simulink model "STmodel_gui"  (R2021b)
settings: Solver=FixedStepDiscrete  StartTime=0.0  StopTime=stop_time  FixedStep=Ts  MaxStep=Ts  RelTol=1e-6  EnableMultiTasking=on
PostLoadFcn:
  | , if any(exist('dsrtsu_mdlpostloadfcn', 'file') == [2, 3, 6]), try dsrtsu_mdlpostloadfcn('Execute', bdroot); catch fprintf('Error in PostLoadFcn (dsrtsu_mdlpostloadfcn) for model "%s":\n %s\n', bdroot, lasterr); end, end,
model workspace (MAT data in the model file):
  Tmp = Simulink.Parameter
  Tmp.Value = Simulink.data.Expression
  Tmp.Value.ExpressionString = "get_param(bdroot,'SimulationTime')"
  Tmp.DataType = 'auto'
  Tmp.Complexity = 'real'
  Tmp.Dimensions = -1
values from neighbouring files (symbols this model uses):
  Cf = 10e-6    (= 1e-05)    [init_STsetup.m]
  fc = 1/Ts    (= 1000)    [init_STsetup.m]
  Filter_d = c2d(Filter,Ts,'Tustin')    [init_STsetup.m]
  fref_st = 50    [init_STsetup.m]
  kii_ST = 250    [init_STsetup.m]
  kiv = 250    [init_STsetup.m]
  kpi_ST = 1.25    [init_STsetup.m]
  kpv = 0.2    [init_STsetup.m]
  Kqload = 2    [init_STsetup.m]
  Lc = 1e-3    (= 0.001)    [init_STsetup.m]
  LoadCurtailment = 0.9    [init_STsetup.m]
  LoadShedding = 0    [init_STsetup.m]
  log_time = 0.2    [init_STsetup.m]
  Pnom = 50e3    (= 50000)    [init_STsetup.m]
  Rc = 0.1    [init_STsetup.m]
  Rf = 2    [init_STsetup.m]
  STstartz = c2d(STstart,Ts,'Tustin')    [init_STsetup.m]
  Ts = 1e-3    (= 0.001)    [init_STsetup.m]
  Vdc = 650    [init_STsetup.m]
  Vref = 325    [init_STsetup.m]
undefined symbols (not defined in the file or in its folder): DiscIntNeverNeededParam
libraries: simulink x4, spsControlledVoltageSourceLib x3, spsThreePhaseSeriesRLCBranchLib x2, spsGroundLib x1, spsRMSLib x1, spsThreePhaseDynamicLoadLib x1, spsThreePhaseVIMeasurementLib x1, spspowerguiLib x1
(part 1 of 2)
settings Model: DSRTSU_INTERNAL_RTI_VER=480  DSRTSU_INTERNAL_RTI_TYPE=rti1006  DSRTSU_INTERNAL_RTIFPGA=70  TunableVars=COMP_GAIN,CurrentLoop,EN_AD,EN_COMPENSATION,EN_DG,EN_ST,FFselection,FREQ_ON,Iref,LEFcontrol,LoadCurtailment,LoadShedding,PLL_Tsettle,P_DG,Q_DG,RST_DG,RST_ST,RSTanalog,VARF,VARV,Vref,calibrationDC_en,calibration_en,fref_st,kc,kii,kii_ST,kiv,kpi,kpi_ST,kpv,krci,krcv,krv  TunableVarsStorageClass=Auto,Auto,Auto,Auto,Auto,Auto,Auto,Auto,Auto,Auto,Auto,Auto,Auto,Auto,Auto,Auto,Auto,Auto,Auto,Auto,Auto,Auto,Auto,Auto,Auto,Auto,Auto,Auto,Auto,Auto,Auto,Auto,Auto,Auto  TunableVarsTypeQualifier=,,,,,,,,,,,,,,,,,,,,,,,,,,,,,,,,,  Creator=zz  LastModifiedBy=bela
settings SolverCC: ConcurrentTasks=on  AlgebraicLoopSolver=TrustRegion  AutoInsertRateTranBlk=on
settings DataIOCC: LimitDataPoints=on  SaveFormat=StructureWithTime  ReturnWorkspaceOutputs=off
settings OptimizationCC: BlockReduction=off  DefaultParameterBehavior=Inlined  EnhancedBackFolding=on  PassReuseOutputArgsAs=Individual arguments  ZeroExternalMemoryAtStartup=off  ZeroInternalMemoryAtStartup=off  OptimizeBlockOrder=speed  DifferentSizesBufferReuse=on  OptimizationCustomize=off  EfficientTunableParamExpr=on
settings DebuggingCC: SolverPrmCheckMsg=warning  ParameterTunabilityLossMsg=error  SFUnexpectedBacktrackingDiag=warning  SFNoUnconditionalDefaultTransitionDiag=warning  SFMachineParentedDataDiag=warning  ArithmeticOperatorsInVariantConditions=warning
settings HardwareCC: ProdBitPerPointer=32  ProdBitPerSizeT=32  ProdBitPerPtrDiffT=32  ProdLargestAtomicFloat=None  ProdWordSize=32  ProdLongLongMode=on  ProdHWDeviceType=Generic->32-bit x86 compatible  TargetBitPerLong=64  TargetBitPerPointer=64  TargetBitPerSizeT=64  TargetBitPerPtrDiffT=64  TargetLongLongMode=on  TargetIntDivRoundTo=Zero  TargetEndianess=LittleEndian  TargetWordSize=64  TargetHWDeviceType=MATLAB Host  ProdEqTarget=off
settings ModelReferenceCC: PropagateSignalLabelsOutOfModel=off
settings SFSimCC: SimUseLocalCustomCode=off  MATLABDynamicMemAlloc=off  CustomCodeUndefinedFunction=UseInterfaceOnly
settings RTWCC: Description=Embedded Coder  SystemTargetFile=ert.tlc  TemplateMakefile=ert_default_tmf  RTWUseLocalCustomCode=off  CodeExecutionProfiling=on  RTWCompilerOptimization=on  CheckMdlBeforeBuild=Warning
settings CodeAppCC: ForceParamTrailComments=on  IgnoreCustomStorageClasses=off  OperatorAnnotations=on  SimulinkDataObjDesc=on  SFDataObjDesc=on  InsertBlockDesc=on
settings ERTTargetCC: TargetLangStandard=C99 (ISO)  GenerateSampleERTMain=on  SupportNonInlinedSFcns=on  InlinedParameterPlacement=NonHierarchical  TargetOS=NativeThreadsExample  ERTCustomFileTemplate=example_file_process.tlc
settings ConfigComp: CovMetricSettings=dw  CovSaveCumulativeToWorkspaceVar=on  CovSaveSingleToWorkspaceVar=on  CovExternalEMLEnable=off  CovSFcnEnable=off

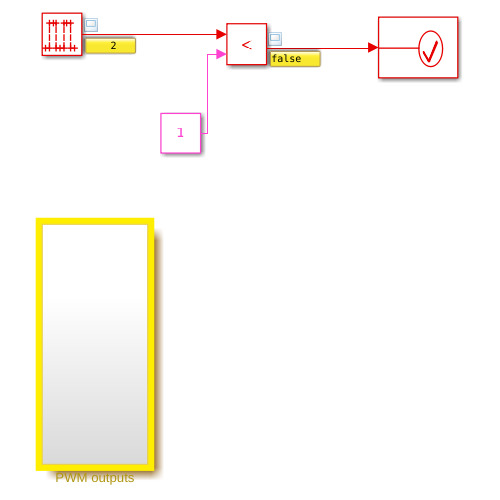
[thumbnail: Simulink's stored preview of the top-level diagram]
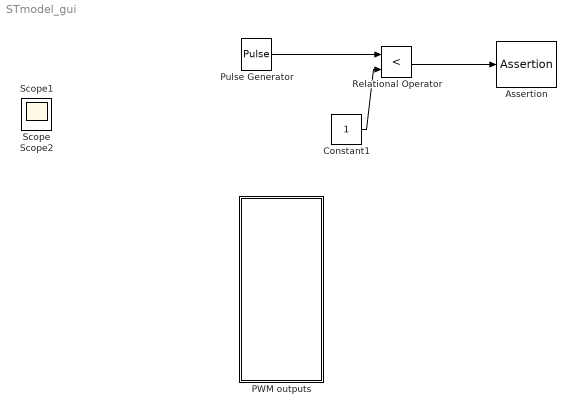
== system STmodel_gui ==
  Assertion : Assertion  AssertionFailFcn=set_param(bdroot,'SimulationCommand','pause')  StopWhenAssertionFail=off
  Constant1 : Constant
  PWM outputs : Subsystem
  Pulse Generator : DiscretePulseGenerator  Amplitude=2  Period=floor(log_time/Ts)  SampleTime=Ts
  Relational Operator : RelationalOperator  Operator=<  OutDataTypeStr=boolean  RndMeth=Simplest
  Scope : Scope
  Scope1 : Scope
  Scope2 : Scope
  wires:
  Constant1/1 -> Relational Operator/2
  Relational Operator/1 -> Assertion/1
  Pulse Generator/1 -> Relational Operator/1

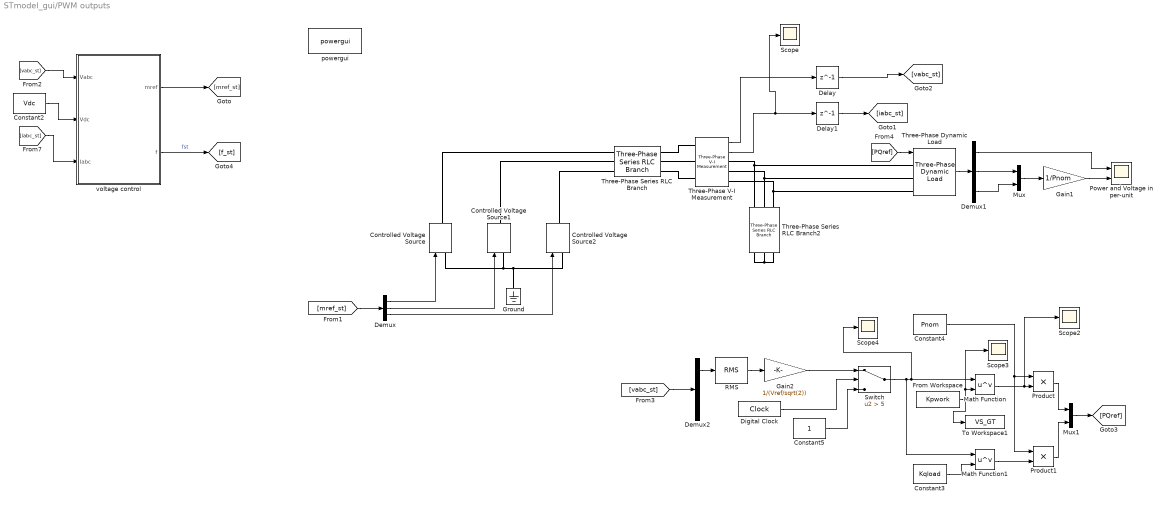
== system STmodel_gui/PWM outputs ==
  Constant2 : Constant  Value=Vdc
  Constant3 : Constant  Value=Kqload
  Constant4 : Constant  Value=Pnom
  Constant5 : Constant
  Controlled Voltage Source : spsControlledVoltageSourceLib/Controlled Voltage Source  Initialize=on  Source_Type=AC  Amplitude=0  Phase=0  Frequency=0  Measurements=None
  Controlled Voltage Source1 : spsControlledVoltageSourceLib/Controlled Voltage Source  Initialize=on  Source_Type=AC  Amplitude=0  Phase=0  Frequency=0  Measurements=None
  Controlled Voltage Source2 : spsControlledVoltageSourceLib/Controlled Voltage Source  Initialize=on  Source_Type=AC  Amplitude=0  Phase=0  Frequency=0  Measurements=None
  Delay : Delay  DelayLength=1  InitialCondition=0
  Delay1 : Delay  DelayLength=1  InitialCondition=0
  Demux : Demux  Outputs=3
  Demux1 : Demux  Outputs=3
  Demux2 : Demux  Outputs=3
  Digital Clock : DigitalClock  SampleTime=Ts
  From Workspace : FromWorkspace  VariableName=Kpwork  OutDataTypeStr=double  SampleTime=-1
  Gain1 : Gain  Gain=1/Pnom
  Gain2 : Gain  Gain=1/(Vref/sqrt(2))
  Ground : spsGroundLib/Ground  LConnTagsString=a
  Math Function : Math  Operator=pow  SaturateOnIntegerOverflow=on
  Math Function1 : Math  Operator=pow  SaturateOnIntegerOverflow=on
  Mux : Mux  Inputs=2
  Mux1 : Mux  Inputs=2
  Power and Voltage in per-unit : Scope  NumInputPorts=2
  Product : Product
  Product1 : Product
  RMS : spsRMSLib/RMS  TrueRMS=on  Freq=50  RMSInit=230  Ts=Ts
  Scope{,2..4} (4 alike) : Scope
  Switch : Switch  Criteria=u2 > Threshold  Threshold=5
  Three-Phase Dynamic Load : spsThreePhaseDynamicLoadLib/Three-Phase Dynamic Load  NominalVoltage=[ 325/sqrt(2)*sqrt(3) 50 ]  ActiveReactivePowers=[50e3 0]  PositiveSequence=[1 0]  ExternalControl=on  NpNq=[1.3 2]  TimeConstants="[0  0  0  0]"  MinimumVoltage=0.7  Tfilter=1e-4  LoadFlowParameters=[4,0,0,0,0]
      settings: SourceProductBaseCode=PS
  Three-Phase Series RLC Branch : spsThreePhaseSeriesRLCBranchLib/Three-Phase Series RLC Branch  LConnTagsString=A|B|C  RConnTagsString=A|B|C  BranchType=RL  Resistance=Rc  Inductance=Lc  Capacitance=1e-6  Measurements=None
  Three-Phase Series RLC Branch2 : spsThreePhaseSeriesRLCBranchLib/Three-Phase Series RLC Branch  LConnTagsString=A|B|C  RConnTagsString=A|B|C  BranchType=RC  Resistance=Rf  Inductance=Lc  Capacitance=Cf  Measurements=None
  Three-Phase V-I Measurement : spsThreePhaseVIMeasurementLib/Three-Phase V-I Measurement  VoltageMeasurement=phase-to-ground  SetLabelV=off  LabelV=Vabc  Vpu=off  VpuLL=off  CurrentMeasurement=yes  SetLabelI=off  LabelI=Iabc  Ipu=off  Pbase=100e6  Vbase=Vref*sqrt(3)/sqrt(2)  OutputType=Complex  PhasorSimulation=off  PSBequivalent=0
  To Workspace1 : ToWorkspace  VariableName=VS_GT  SampleTime=log_time
      settings: MaxDataPoints=floor(log_time/Ts)  Save2DSignal=2-D array (concatenate along first dimension)
  powergui : spspowerguiLib/powergui  Priority=1  SimulationMode=Discrete  SampleTime=Ts  frequency=60  Iterations=50  frequencyindice=0  Pbase=100e6  ErrMax=1e-4  UnitsV=kV  UnitsW=MW  buscounter=0  FunctionMessages=off  echomessages=off  EnableUseOfTLC=off  CurrentSourceSwitches=off  DisableSnubberDevices=off  DisableRonSwitches=off  DisableVfSwitches=off  DisplayEquations=off  AutomaticDiscreteSolvers=off  SolverType=Tustin/Backward Euler (TBE)  Interpol=off  ExternalGateDelay=off  methode=off  Ts=100  x0status=blocks  SPID=on  SwTol=0  HookPort=off  NonlinearTolerance=1e-4  nMaxIteration=100  ContinueOnMaxIteration=off  RestoreLinks=warning  ResistiveCurrentMeasurement=off  Frange=[0:2:500]  Ylog=off  Xlog=on  ShowGrid=off  save=off  variable=ZData  structure=0  ZoomFFT=off  StartTime=0.0  cycles=1  DisplayStyle=1  fundamental=60  FreqAxis=off  MaxFrequency=1000  frequencyindicesteady=1  RmsSteady=1  display=off
  voltage control : Subsystem
  wires:
  voltage control/1(mref) -> [mref_st]
  [vabc_st] -> voltage control/1(Vabc)
  Constant2/1 -> voltage control/2(Vdc)
  [iabc_st] -> voltage control/3(Iabc)
  voltage control/2(f) -> [f_st]  "fst"
  [mref_st] -> Demux/1
  Demux/3 -> Controlled Voltage Source2/1
  Demux/2 -> Controlled Voltage Source1/1
  Demux/1 -> Controlled Voltage Source/1
  Three-Phase V-I Measurement/2 -> Scope/1, Delay1/1
  Three-Phase V-I Measurement/1 -> Delay/1
  Delay/1 -> [vabc_st]
  Delay1/1 -> [iabc_st]
  Demux1/1 -> Power and Voltage in per-unit/1
  Demux1/2 -> Mux/1
  Demux1/3 -> Mux/2
  Mux/1 -> Gain1/1
  Gain1/1 -> Power and Voltage in per-unit/2
  RMS/1 -> Gain2/1
  Switch/1 -> Math Function1/1, Scope4/1, Math Function/1
  From Workspace/1 -> To Workspace1/1, Scope3/1, Math Function/2
  Constant3/1 -> Math Function1/2
  Math Function/1 -> Scope2/1, Product/2
  Math Function1/1 -> Product1/2
  Constant4/1 -> Product1/1, Product/1
  Mux1/1 -> [PQref]
  Product/1 -> Mux1/1
  Product1/1 -> Mux1/2
  [vabc_st] -> Demux2/1
  Gain2/1 -> Switch/1
  Constant5/1 -> Switch/3
  Digital Clock/1 -> Switch/2
  Three-Phase Dynamic Load/1 -> Demux1/1
  [PQref] -> Three-Phase Dynamic Load/1
  Demux2/1 -> RMS/1
  connections:
  Controlled Voltage Source/LConn1 -- Ground/LConn1 -- Controlled Voltage Source2/LConn1 -- Controlled Voltage Source1/LConn1
  Three-Phase Series RLC Branch2/RConn1 -- Three-Phase Series RLC Branch2/RConn3 -- Three-Phase Series RLC Branch2/RConn2
  Three-Phase Series RLC Branch/LConn1 -- Controlled Voltage Source/RConn1
  Three-Phase Series RLC Branch/LConn2 -- Controlled Voltage Source1/RConn1
  Three-Phase Series RLC Branch/LConn3 -- Controlled Voltage Source2/RConn1
  Three-Phase V-I Measurement/LConn2 -- Three-Phase Series RLC Branch/RConn2
  Three-Phase Series RLC Branch/RConn1 -- Three-Phase V-I Measurement/LConn1
  Three-Phase Series RLC Branch/RConn3 -- Three-Phase V-I Measurement/LConn3
  Three-Phase V-I Measurement/RConn1 -- Three-Phase Dynamic Load/LConn1 -- Three-Phase Series RLC Branch2/LConn1
  Three-Phase V-I Measurement/RConn2 -- Three-Phase Dynamic Load/LConn2 -- Three-Phase Series RLC Branch2/LConn2
  Three-Phase V-I Measurement/RConn3 -- Three-Phase Dynamic Load/LConn3 -- Three-Phase Series RLC Branch2/LConn3

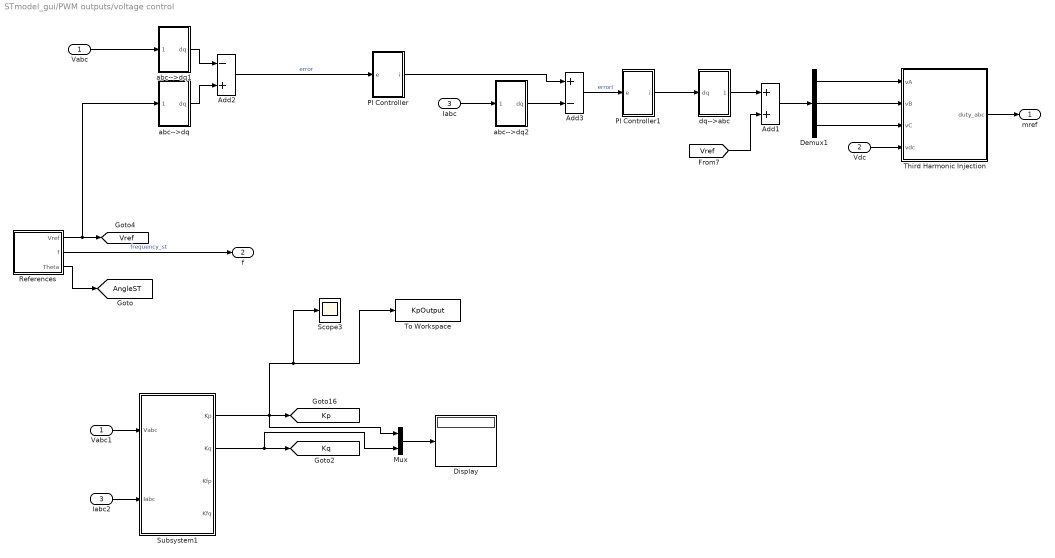
== system STmodel_gui/PWM outputs/voltage control ==
  Vabc : Inport
  Vdc : Inport  Port=2
  Iabc : Inport  Port=3
  Add1 : Sum
  Add2 : Sum  Inputs=-+
  Add3 : Sum  Inputs=+-
  Demux1 : Demux  Outputs=3
  Display : Display
  Iabc2 : InportShadow  Port=3
  Mux : Mux  Inputs=2
  PI Controller : Subsystem
  PI Controller1 : Subsystem
  References : Subsystem
  Scope3 : Scope
  Subsystem1 : Subsystem
  Third Harmonic Injection : Subsystem
      mask Display: disp('Modulation');
  To Workspace : ToWorkspace  VariableName=KpOutput  SampleTime=log_time
      settings: MaxDataPoints=floor(log_time/Ts)  Save2DSignal=2-D array (concatenate along first dimension)
  Vabc1 : InportShadow
  abc-->dq : Subsystem
  abc-->dq1 : Subsystem
  abc-->dq2 : Subsystem
  dq-->abc : Subsystem
  mref : Outport
  f : Outport  Port=2
  tag scope: AngleST=global, Kp=global, Kq=global, Vref=global
  wires:
  [Vref] -> Add1/2
  Vabc1/1 -> Subsystem1/1(Vabc)
  Iabc2/1 -> Subsystem1/2(Iabc)
  Subsystem1/2(Kq) -> Mux/2, [Kq]
  Subsystem1/1(Kp) -> Scope3/1, To Workspace/1, Mux/1, [Kp]
  Demux1/3 -> Third Harmonic Injection/3(vC)
  Demux1/2 -> Third Harmonic Injection/2("vB ")
  Demux1/1 -> Third Harmonic Injection/1(vA)
  Add2/1 -> PI Controller/1(e)  "error"
  Vabc/1 -> abc-->dq1/1(abc)
  References/2(f) -> f/1  "frequency_st"
  References/1(Vref) -> abc-->dq/1(abc), [Vref]
  Vdc/1 -> Third Harmonic Injection/4(vdc)
  Third Harmonic Injection/1(duty_abc) -> mref/1
  Iabc/1 -> abc-->dq2/1(abc)
  Add3/1 -> PI Controller1/1(e)  "errorI"
  abc-->dq2/1(dq) -> Add3/2
  References/3(Theta) -> [AngleST]
  abc-->dq/1(dq) -> Add2/2
  abc-->dq1/1(dq) -> Add2/1
  PI Controller1/1(i) -> dq-->abc/1(dq)
  dq-->abc/1(abc) -> Add1/1
  PI Controller/1(i) -> Add3/1
  Mux/1 -> Display/1
  Add1/1 -> Demux1/1

== system STmodel_gui/PWM outputs/voltage control/PI Controller ==
  e : Inport
  Demux : Demux  Outputs=2
  Mux1 : Mux  Inputs=2
  Subsystem1 : Subsystem
  Subsystem2 : Subsystem
  i : Outport
  wires:
  Mux1/1 -> i/1
  Subsystem2/1(out) -> Mux1/2
  Subsystem1/1(out) -> Mux1/1
  Demux/2 -> Subsystem2/1(e)
  Demux/1 -> Subsystem1/1(e)
  e/1 -> Demux/1

== system STmodel_gui/PWM outputs/voltage control/PI Controller1 ==
  e : Inport
  Demux : Demux  Outputs=2
  Mux1 : Mux  Inputs=2
  Subsystem1 : Subsystem
  Subsystem2 : Subsystem
  i : Outport
  wires:
  e/1 -> Demux/1
  Demux/1 -> Subsystem1/1(e)
  Demux/2 -> Subsystem2/1(e)
  Subsystem1/1(out) -> Mux1/1
  Subsystem2/1(out) -> Mux1/2
  Mux1/1 -> i/1

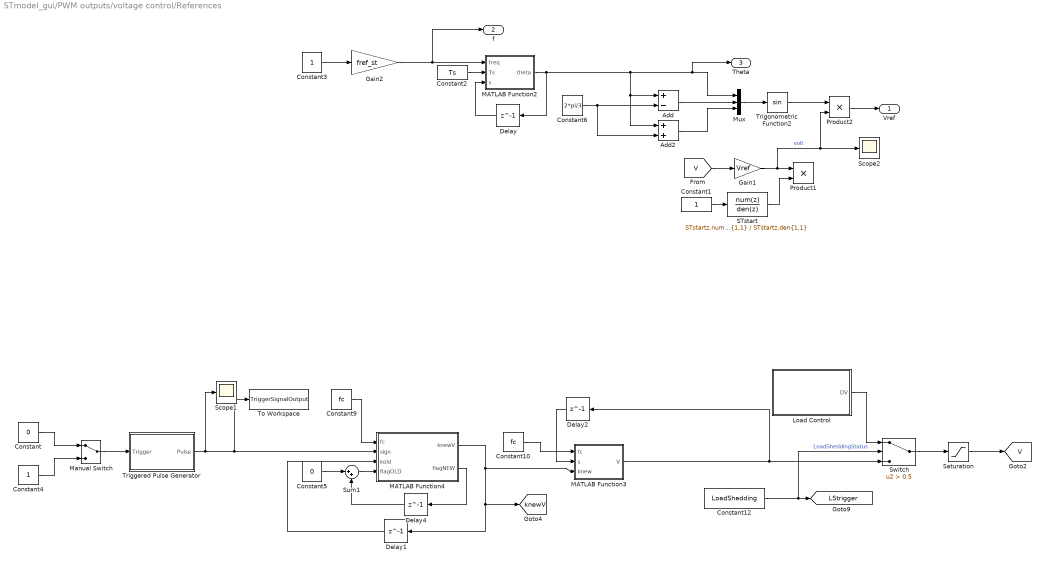
== system STmodel_gui/PWM outputs/voltage control/References ==
  Add : Sum  Inputs=+-
  Add2 : Sum
  Constant : Constant  Value=0
  Constant1 : Constant
  Constant10 : Constant  Value=fc
  Constant12 : Constant  Value=LoadShedding
  Constant2 : Constant  Value=Ts
  Constant3 : Constant
  Constant4 : Constant
  Constant5 : Constant  Value=0
  Constant6 : Constant  Value=2*pi/3
  Constant9 : Constant  Value=fc
  Delay{,1..2,4} (4 alike) : Delay  DelayLength=1  InitialCondition=0
  Gain1 : Gain  Gain=Vref
  Gain2 : Gain  Gain=fref_st
  Load Control : Subsystem
  MATLAB Function2 : MATLAB Function  TreatAsAtomicUnit=on
  MATLAB Function3 : MATLAB Function  TreatAsAtomicUnit=on
  MATLAB Function4 : MATLAB Function  TreatAsAtomicUnit=on
  Manual Switch : ManualSwitch
  Mux : Mux  Inputs=3
  Product1 : Product
  Product2 : Product
  STstart : DiscreteFilter  Numerator=STstartz.num{1,1}  Denominator=STstartz.den{1,1}
  Saturation : Saturate  UpperLimit=1.1  LowerLimit=0.85
  Scope1 : Scope
  Scope2 : Scope
  Sum1 : Sum  Inputs=|++
  Switch : Switch  Criteria=u2 > Threshold  Threshold=0.5
  To Workspace : ToWorkspace  VariableName=TriggerSignalOutput  SampleTime=log_time
      settings: MaxDataPoints=floor(log_time/Ts)  Save2DSignal=2-D array (concatenate along first dimension)
  Triggered Pulse Generator : Subsystem  TreatAsAtomicUnit=on  mask(single pulse generation){p_wid=2000}
      mask prompts: p_wid "pulse width (number of samples)"
      mask help: This block generate a single pulse whenever a trigger happen. The pulse width must specified as a number of samples. for example if your sampling time is 0.1s and you want 3s pulse , then you should enter 30 as a pulse width.
      mask Display:
      | plot([0],[0])
      | plot([11],[0])
      | plot([5],[0.5])
      | plot([4 5 5 6 6 7],[0 0 0.25 0.25 0 0])
      | plot([5],[-0.3])
      | 
      | port_label('output', 1, 'Pulse')
      | port_label('input', 1, 'Trigger')
  Trigonometric Function2 : Trigonometry
  Vref : Outport
  f : Outport  Port=2
  Theta : Outport  Port=3
  tag scope: LStrigger=global, V=global, knewV=global
  wires:
  Saturation/1 -> [V]
  Switch/1 -> Saturation/1
  MATLAB Function3/1(V) -> Switch/3, Delay2/1
  Constant12/1 -> [LStrigger], Switch/2  "LoadSheddingStatus"
  Constant10/1 -> MATLAB Function3/1(fc)
  Constant9/1 -> MATLAB Function4/1(fc)
  Delay4/1 -> Sum1/2
  MATLAB Function4/2(flagNEW) -> Delay4/1
  Sum1/1 -> MATLAB Function4/4(flagOLD)
  Constant5/1 -> Sum1/1
  Delay1/1 -> MATLAB Function4/3(kold)
  MATLAB Function4/1(knewV) -> MATLAB Function3/3(knew), Delay1/1, [knewV]
  Delay2/1 -> MATLAB Function3/2(s)
  Product2/1 -> Vref/1
  Mux/1 -> Trigonometric Function2/1
  MATLAB Function2/1(theta) -> Theta/1, Mux/1, Add/1, Add2/1, Delay/1
  Constant6/1 -> Add2/2, Add/2
  Add/1 -> Mux/2
  Add2/1 -> Mux/3
  Delay/1 -> MATLAB Function2/3(s)
  Trigonometric Function2/1 -> Product2/1
  Gain2/1 -> MATLAB Function2/1(freq), f/1
  [V] -> Gain1/1
  Constant3/1 -> Gain2/1
  Constant2/1 -> MATLAB Function2/2(Ts)
  Gain1/1 -> Scope2/1, Product2/2, Product1/1  "volt"
  Constant1/1 -> STstart/1
  STstart/1 -> Product1/2
  Load Control/1(DV) -> Switch/1
  Constant4/1 -> Manual Switch/2
  Constant/1 -> Manual Switch/1
  Manual Switch/1 -> Triggered Pulse Generator/1(Trigger)
  Triggered Pulse Generator/1(Pulse) -> Scope1/1, MATLAB Function4/2(sign), To Workspace/1

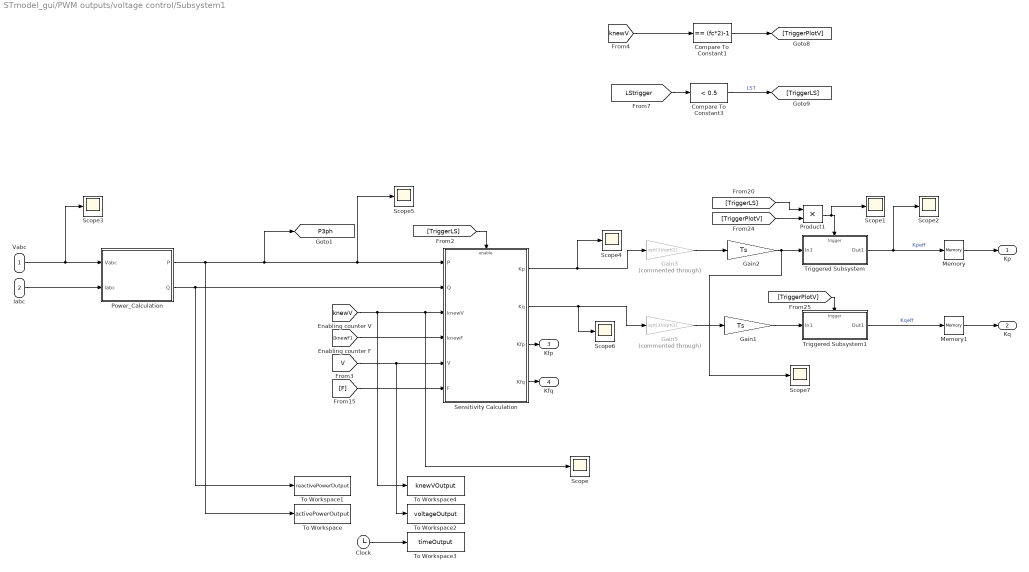
== system STmodel_gui/PWM outputs/voltage control/Subsystem1 ==
  Vabc : Inport
  Iabc : Inport  Port=2
  Clock : Clock
  Compare To Constant1 : simulink/Logic and Bit Operations/Compare To Constant  relop===  const=(fc*2)-1  OutDataTypeStr=boolean
  Compare To Constant3 : simulink/Logic and Bit Operations/Compare To Constant  relop=<  const=0.5  OutDataTypeStr=boolean
  Gain1 : Gain  Gain=Ts
  Gain2 : Gain  Gain=Ts
  Gain3 : Gain  Commented=through  Gain=sqrt(3)/sqrt(2)
  Gain5 : Gain  Commented=through  Gain=sqrt(3)/sqrt(2)
  Memory : Memory  InitialCondition=1  InheritSampleTime=on
  Memory1 : Memory  InheritSampleTime=on
  Power_Calculation : Subsystem
  Product1 : Product
  Scope{,1..7} (8 alike) : Scope
  Sensitivity Calculation : Subsystem  TreatAsAtomicUnit=on
  To Workspace : ToWorkspace  VariableName=activePowerOutput  SampleTime=log_time
      settings: MaxDataPoints=floor(log_time/Ts)  Save2DSignal=2-D array (concatenate along first dimension)
  To Workspace1 : ToWorkspace  VariableName=reactivePowerOutput  SampleTime=log_time
      settings: MaxDataPoints=floor(log_time/Ts)  Save2DSignal=2-D array (concatenate along first dimension)
  To Workspace2 : ToWorkspace  VariableName=voltageOutput  SampleTime=log_time
      settings: MaxDataPoints=floor(log_time/Ts)  Save2DSignal=2-D array (concatenate along first dimension)
  To Workspace3 : ToWorkspace  VariableName=timeOutput  SampleTime=log_time
      settings: MaxDataPoints=floor(log_time/Ts)  Save2DSignal=2-D array (concatenate along first dimension)
  To Workspace4 : ToWorkspace  VariableName=knewVOutput  SampleTime=log_time
      settings: MaxDataPoints=floor(log_time/Ts)  Save2DSignal=2-D array (concatenate along first dimension)
  Triggered Subsystem : Subsystem  TreatAsAtomicUnit=on
  Triggered Subsystem1 : Subsystem  TreatAsAtomicUnit=on
  Kp : Outport
  Kq : Outport  Port=2
  Kfp : Outport  Port=3
  Kfq : Outport  Port=4
  tag scope: P3ph=global
  wires:
  Sensitivity Calculation/4(Kfq) -> Kfq/1
  Sensitivity Calculation/3(Kfp) -> Kfp/1
  Gain2/1 -> Scope7/1, Triggered Subsystem/1(In1)
  [TriggerPlotV] -> Triggered Subsystem1/Trigger
  Triggered Subsystem/1(Out1) -> Scope2/1, Memory/1  "Kpeff"
  Triggered Subsystem1/1(Out1) -> Memory1/1  "Kqeff"
  Gain1/1 -> Triggered Subsystem1/1(In1)
  Sensitivity Calculation/2(Kq) -> Scope6/1, Gain5/1
  [knewV] -> Compare To Constant1/1
  Compare To Constant1/1 -> [TriggerPlotV]
  [knewV] -> To Workspace4/1, Scope/1, Sensitivity Calculation/3(knewV)
  [knewF] -> Sensitivity Calculation/4(knewF)
  [V] -> To Workspace2/1, Sensitivity Calculation/5(V)
  [F] -> Sensitivity Calculation/6(F)
  Memory/1 -> Kp/1
  [LStrigger] -> Compare To Constant3/1
  Compare To Constant3/1 -> [TriggerLS]  "LST"
  [TriggerLS] -> Sensitivity Calculation/Enable
  [TriggerPlotV] -> Product1/2
  [TriggerLS] -> Product1/1
  Product1/1 -> Scope1/1, Triggered Subsystem/Trigger
  Memory1/1 -> Kq/1
  Power_Calculation/1(P) -> To Workspace/1, Sensitivity Calculation/1(P), Scope5/1, [P3ph]
  Vabc/1 -> Scope3/1, Power_Calculation/1(Vabc)
  Iabc/1 -> Power_Calculation/2(Iabc)
  Gain3/1 -> Gain2/1
  Gain5/1 -> Gain1/1
  Power_Calculation/2(Q) -> To Workspace1/1, Sensitivity Calculation/2(Q)
  Clock/1 -> To Workspace3/1
  Sensitivity Calculation/1(Kp) -> Scope4/1, Gain3/1

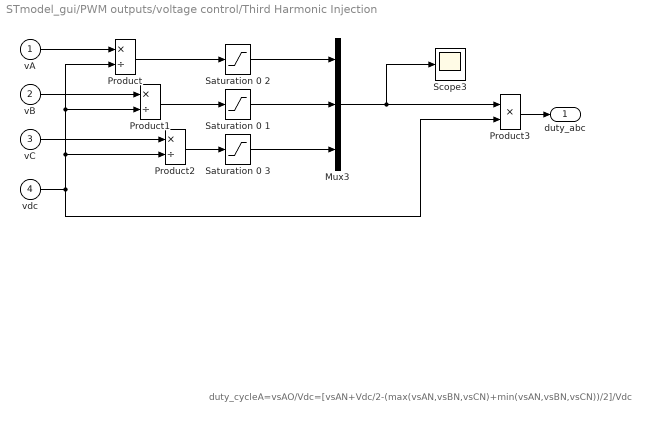
== system STmodel_gui/PWM outputs/voltage control/Third Harmonic Injection ==
  note: duty_cycleA=vsAO/Vdc=[vsAN+Vdc/2-(max(vsAN,vsBN,vsCN)+min(vsAN,vsBN,vsCN))/2]/Vdc
  vA : Inport
  "vB " : Inport  Port=2
  vC : Inport  Port=3
  vdc : Inport  Port=4
  Mux3 : Mux  Inputs=3
  Product : Product  Inputs=*/  SaturateOnIntegerOverflow=on  OutDataTypeStr=Inherit: Same as first input
  Product1 : Product  Inputs=*/  SaturateOnIntegerOverflow=on  OutDataTypeStr=Inherit: Same as first input
  Product2 : Product  Inputs=*/  SaturateOnIntegerOverflow=on  OutDataTypeStr=Inherit: Same as first input
  Product3 : Product  Inputs=**  SaturateOnIntegerOverflow=on  OutDataTypeStr=Inherit: Same as first input
  Saturation 0 1 : Saturate  UpperLimit=1  LowerLimit=-1
  Saturation 0 2 : Saturate  UpperLimit=1  LowerLimit=-1
  Saturation 0 3 : Saturate  UpperLimit=1  LowerLimit=-1
  Scope3 : Scope
  duty_abc : Outport
  wires:
  Product2/1 -> Saturation 0 3/1
  "vB "/1 -> Product1/1
  vdc/1 -> Product3/2, Product2/2, Product1/2, Product/2
  Product1/1 -> Saturation 0 1/1
  Product/1 -> Saturation 0 2/1
  Saturation 0 3/1 -> Mux3/3
  Saturation 0 1/1 -> Mux3/2
  Saturation 0 2/1 -> Mux3/1
  vA/1 -> Product/1
  vC/1 -> Product2/1
  Mux3/1 -> Scope3/1, Product3/1
  Product3/1 -> duty_abc/1

== system STmodel_gui/PWM outputs/voltage control/abc-->dq ==
  abc : Inport
  alpha,beta --> d,q1 : Subsystem
  clarke3 : Gain  Gain=(2/3)*[1 -0.5 -0.5; 0 sqrt(3)/2 -sqrt(3)/2]  Multiplication=Matrix(K*u)
  dq : Outport
  wires:
  alpha,beta --> d,q1/1(d,q) -> dq/1
  clarke3/1 -> alpha,beta --> d,q1/1("alpha, beta")
  [AngleST] -> alpha,beta --> d,q1/2(phi)
  abc/1 -> clarke3/1

== system STmodel_gui/PWM outputs/voltage control/abc-->dq1 ==
  abc : Inport
  alpha,beta --> d,q : Subsystem
  clarke2 : Gain  Gain=(2/3)*[1 -0.5 -0.5; 0 sqrt(3)/2 -sqrt(3)/2]  Multiplication=Matrix(K*u)
  dq : Outport
  wires:
  alpha,beta --> d,q/1(d,q) -> dq/1  "vref"
  clarke2/1 -> alpha,beta --> d,q/1("alpha, beta")  "vref"
  [AngleST] -> alpha,beta --> d,q/2(phi)
  abc/1 -> clarke2/1

== system STmodel_gui/PWM outputs/voltage control/abc-->dq2 ==
  abc : Inport
  alpha,beta --> d,q1 : Subsystem
  clarke3 : Gain  Gain=(2/3)*[1 -0.5 -0.5; 0 sqrt(3)/2 -sqrt(3)/2]  Multiplication=Matrix(K*u)
  dq : Outport
  wires:
  abc/1 -> clarke3/1
  [AngleST] -> alpha,beta --> d,q1/2(phi)
  clarke3/1 -> alpha,beta --> d,q1/1("alpha, beta")
  alpha,beta --> d,q1/1(d,q) -> dq/1

== system STmodel_gui/PWM outputs/voltage control/dq-->abc ==
  dq : Inport
  alpha,beta --> d,q3 : Subsystem
  clarke : Gain  Gain=[1 0; -0.5 sqrt(3)/2; -0.5 -sqrt(3)/2]  Multiplication=Matrix(K*u)
  abc : Outport
  wires:
  dq/1 -> alpha,beta --> d,q3/1("d, q")
  alpha,beta --> d,q3/1("alfa, beta") -> clarke/1
  [AngleST] -> alpha,beta --> d,q3/2(phi)
  clarke/1 -> abc/1

== system STmodel_gui/PWM outputs/voltage control/PI Controller/Subsystem1 ==
  e : Inport
  Discrete-Time Integrator : DiscreteIntegrator  SampleTime=-1  LimitOutput=on  UpperSaturationLimit=Vdc  LowerSaturationLimit=-Vdc  ICPrevOutput=DiscIntNeverNeededParam  ICPrevScaledInput=DiscIntNeverNeededParam
  Kp : Gain  Gain=kpv
  Kp1 : Gain  Gain=kiv
  Sum : Sum
  out : Outport
  wires:
  e/1 -> Kp1/1, Kp/1
  Kp1/1 -> Discrete-Time Integrator/1
  Kp/1 -> Sum/1
  Sum/1 -> out/1
  Discrete-Time Integrator/1 -> Sum/2

== system STmodel_gui/PWM outputs/voltage control/PI Controller/Subsystem2 ==
  e : Inport
  Discrete-Time Integrator : DiscreteIntegrator  SampleTime=-1  LimitOutput=on  UpperSaturationLimit=Vdc  LowerSaturationLimit=-Vdc  ICPrevOutput=DiscIntNeverNeededParam  ICPrevScaledInput=DiscIntNeverNeededParam
  Kp : Gain  Gain=kpv
  Kp1 : Gain  Gain=kiv
  Sum : Sum
  out : Outport
  wires:
  Discrete-Time Integrator/1 -> Sum/2
  Sum/1 -> out/1
  Kp/1 -> Sum/1
  Kp1/1 -> Discrete-Time Integrator/1
  e/1 -> Kp/1, Kp1/1

== system STmodel_gui/PWM outputs/voltage control/PI Controller1/Subsystem1 ==
  e : Inport
  Discrete-Time Integrator : DiscreteIntegrator  SampleTime=-1  LimitOutput=on  UpperSaturationLimit=Vdc  LowerSaturationLimit=-Vdc  ICPrevOutput=DiscIntNeverNeededParam  ICPrevScaledInput=DiscIntNeverNeededParam
  Kp : Gain  Gain=kpi_ST
  Kp1 : Gain  Gain=kii_ST
  Sum : Sum
  out : Outport
  wires:
  Discrete-Time Integrator/1 -> Sum/2
  Sum/1 -> out/1
  Kp/1 -> Sum/1
  Kp1/1 -> Discrete-Time Integrator/1
  e/1 -> Kp/1, Kp1/1

== system STmodel_gui/PWM outputs/voltage control/PI Controller1/Subsystem2 ==
  e : Inport
  Discrete-Time Integrator : DiscreteIntegrator  SampleTime=-1  LimitOutput=on  UpperSaturationLimit=Vdc  LowerSaturationLimit=-Vdc  ICPrevOutput=DiscIntNeverNeededParam  ICPrevScaledInput=DiscIntNeverNeededParam
  Kp : Gain  Gain=kpi_ST
  Kp1 : Gain  Gain=kii_ST
  Sum : Sum
  out : Outport
  wires:
  e/1 -> Kp1/1, Kp/1
  Kp1/1 -> Discrete-Time Integrator/1
  Kp/1 -> Sum/1
  Sum/1 -> out/1
  Discrete-Time Integrator/1 -> Sum/2

== system STmodel_gui/PWM outputs/voltage control/References/Load Control ==
  Add1 : Sum
  Add5 : Sum  Inputs=-+
  Constant11 : Constant  Value=LoadCurtailment
  Constant8 : Constant
  Delay5 : Delay  DelayLength=1  InitialCondition=0
  Divide1 : Product  Inputs=*/
  Product4 : Product
  Product7 : Product
  DV : Outport
  wires:
  Constant8/1 -> Add1/1
  Divide1/1 -> Add1/2
  Delay5/1 -> Divide1/2
  Add5/1 -> Divide1/1
  Product4/1 -> Delay5/1
  [Kp] -> Product4/2
  [P3ph] -> Product4/1
  Product7/1 -> Add5/2
  Constant11/1 -> Product7/2
  [P3ph] -> Add5/1, Product7/1
  Add1/1 -> DV/1  "DV"

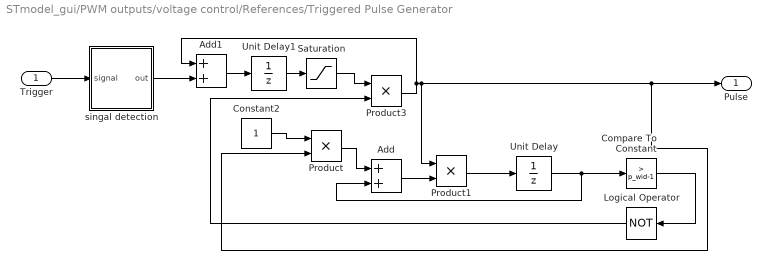
== system STmodel_gui/PWM outputs/voltage control/References/Triggered Pulse Generator ==
  Trigger : Inport
  Add : Sum
  Add1 : Sum
  Compare To Constant : simulink/Logic and Bit Operations/Compare To Constant  relop=>  const=p_wid-1  OutDataTypeStr=boolean
  Constant2 : Constant
  Logical Operator : Logic  Operator=NOT  AllPortsSameDT=off  OutDataTypeStr=boolean
  Product : Product  RndMeth=Zero
  Product1 : Product  RndMeth=Zero
  Product3 : Product  RndMeth=Zero
  Saturation : Saturate  UpperLimit=1  LowerLimit=0
  Unit Delay : UnitDelay  SampleTime=-1  HasFrameUpgradeWarning=on
  Unit Delay1 : UnitDelay  SampleTime=-1  HasFrameUpgradeWarning=on
  singal detection : Subsystem
  Pulse : Outport
  wires:
  Compare To Constant/1 -> Logical Operator/1
  Constant2/1 -> Product/1
  Product/1 -> Add/1
  Unit Delay/1 -> Add/2, Compare To Constant/1
  Trigger/1 -> singal detection/1(signal)
  singal detection/1(out) -> Add1/2
  Add/1 -> Product1/2
  Product1/1 -> Unit Delay/1
  Add1/1 -> Unit Delay1/1
  Unit Delay1/1 -> Saturation/1
  Saturation/1 -> Product3/1
  Product3/1 -> Product/2, Pulse/1, Product1/1, Add1/1
  Logical Operator/1 -> Product3/2

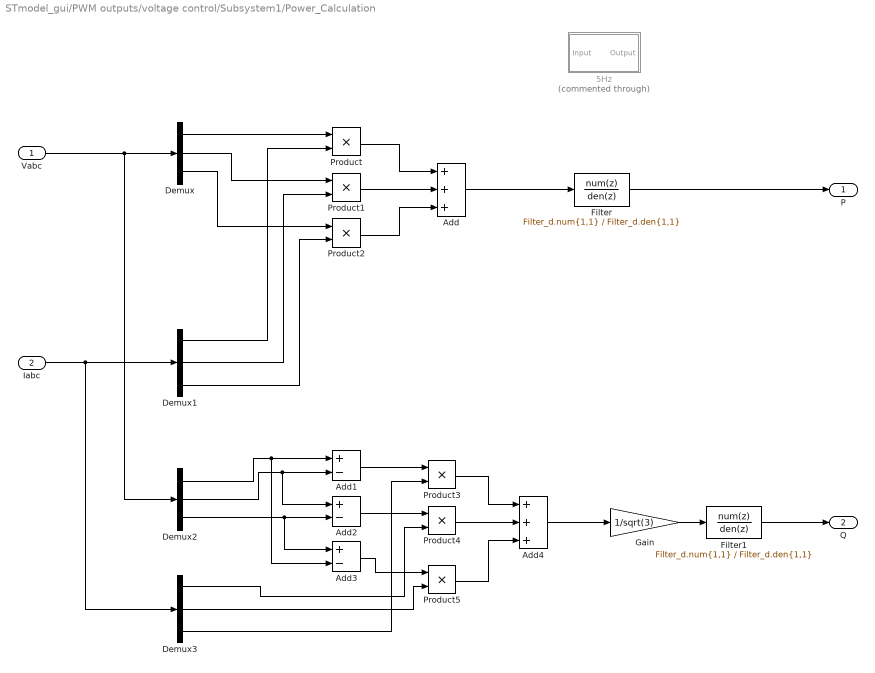
== system STmodel_gui/PWM outputs/voltage control/Subsystem1/Power_Calculation ==
  Vabc : Inport
  Iabc : Inport  Port=2
  5Hz : Subsystem  Tag=FilterWizardSubSystem  Commented=through
      settings: ErrorFcn=dspFilterRealizedInBasicElemsAlgLoopErrFcnCallback
  Add : Sum  Inputs=+++
  Add1 : Sum  Inputs=+-
  Add2 : Sum  Inputs=+-
  Add3 : Sum  Inputs=+-
  Add4 : Sum  Inputs=+++
  Demux{,1..3} (4 alike) : Demux  Outputs=3
  Filter : DiscreteFilter  Numerator=Filter_d.num{1,1}  Denominator=Filter_d.den{1,1}
  Filter1 : DiscreteFilter  Numerator=Filter_d.num{1,1}  Denominator=Filter_d.den{1,1}
  Gain : Gain  Gain=1/sqrt(3)
  Product{,1..5} (6 alike) : Product
  P : Outport
  Q : Outport  Port=2
  wires:
  Vabc/1 -> Demux2/1, Demux/1
  Iabc/1 -> Demux3/1, Demux1/1
  Demux/1 -> Product/1
  Demux/2 -> Product1/1
  Demux/3 -> Product2/1
  Demux1/1 -> Product/2
  Demux1/2 -> Product1/2
  Demux1/3 -> Product2/2
  Product/1 -> Add/1
  Product1/1 -> Add/2
  Product2/1 -> Add/3
  Add/1 -> Filter/1
  Filter/1 -> P/1
  Demux2/1 -> Add3/2, Add1/1
  Demux2/2 -> Add2/1, Add1/2
  Add1/1 -> Product3/1
  Demux3/3 -> Product3/2
  Demux2/3 -> Add3/1, Add2/2
  Add2/1 -> Product4/1
  Demux3/1 -> Product4/2
  Add3/1 -> Product5/1
  Demux3/2 -> Product5/2
  Product4/1 -> Add4/2
  Product3/1 -> Add4/1
  Product5/1 -> Add4/3
  Add4/1 -> Gain/1
  Gain/1 -> Filter1/1
  Filter1/1 -> Q/1

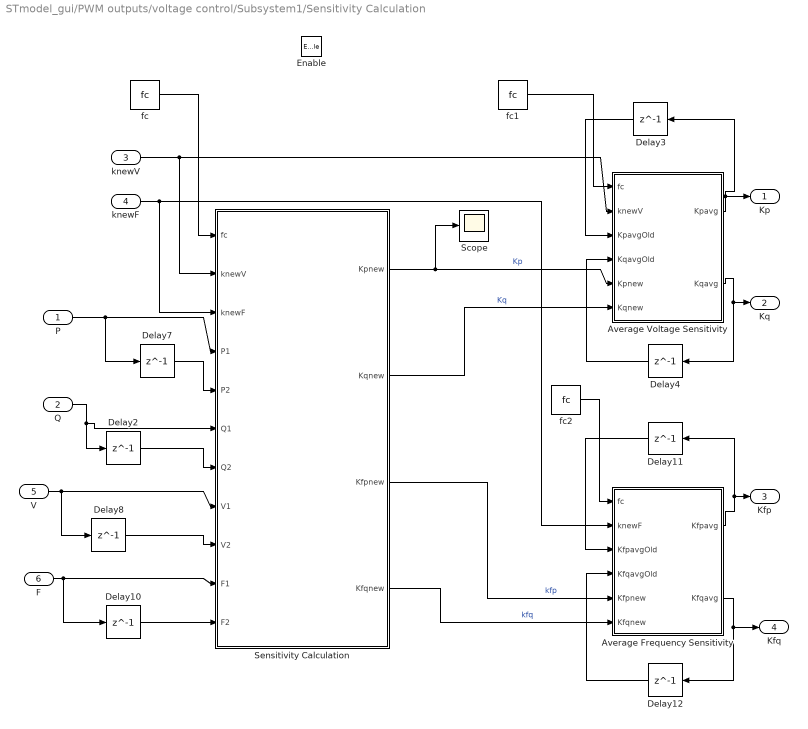
== system STmodel_gui/PWM outputs/voltage control/Subsystem1/Sensitivity Calculation ==
  P : Inport
  Q : Inport  Port=2
  knewV : Inport  Port=3
  knewF : Inport  Port=4
  V : Inport  Port=5
  F : Inport  Port=6
  Enable : EnablePort
  Average Frequency Sensitivity : MATLAB Function  InitFcn=|  TreatAsAtomicUnit=on
      | KpavgOld=0;
      | Kpavg=0;
  Average Voltage Sensitivity : MATLAB Function  InitFcn=|  TreatAsAtomicUnit=on
      | KpavgOld=0;
      | Kpavg=0;
  Delay{2..4,7..8,10..12} (8 alike) : Delay  DelayLength=1  InitialCondition=0
  Scope : Scope
  Sensitivity Calculation : MATLAB Function  TreatAsAtomicUnit=on
  fc : Constant  Value=fc
  fc1 : Constant  Value=fc
  fc2 : Constant  Value=fc
  Kp : Outport
  Kq : Outport  Port=2
  Kfp : Outport  Port=3
  Kfq : Outport  Port=4
  wires:
  Sensitivity Calculation/1(Kpnew) -> Scope/1, Average Voltage Sensitivity/5(Kpnew)  "Kp"
  Delay7/1 -> Sensitivity Calculation/5(P2)
  Delay8/1 -> Sensitivity Calculation/9(V2)
  Average Voltage Sensitivity/1(Kpavg) -> Kp/1, Delay3/1
  Delay3/1 -> Average Voltage Sensitivity/3(KpavgOld)
  Average Voltage Sensitivity/2(Kqavg) -> Kq/1, Delay4/1
  Delay2/1 -> Sensitivity Calculation/7(Q2)
  Sensitivity Calculation/2(Kqnew) -> Average Voltage Sensitivity/6(Kqnew)  "Kq"
  Delay4/1 -> Average Voltage Sensitivity/4(KqavgOld)
  Delay10/1 -> Sensitivity Calculation/11(F2)
  Sensitivity Calculation/3(Kfpnew) -> Average Frequency Sensitivity/5(Kfpnew)  "kfp"
  Average Frequency Sensitivity/1(Kfpavg) -> Kfp/1, Delay11/1
  Delay11/1 -> Average Frequency Sensitivity/3(KfpavgOld)
  Delay12/1 -> Average Frequency Sensitivity/4(KfqavgOld)
  Sensitivity Calculation/4(Kfqnew) -> Average Frequency Sensitivity/6(Kfqnew)  "kfq"
  knewF/1 -> Average Frequency Sensitivity/2(knewF), Sensitivity Calculation/3(knewF)
  knewV/1 -> Sensitivity Calculation/2(knewV), Average Voltage Sensitivity/2(knewV)
  P/1 -> Delay7/1, Sensitivity Calculation/4(P1)
  Q/1 -> Delay2/1, Sensitivity Calculation/6(Q1)
  Average Frequency Sensitivity/2(Kfqavg) -> Kfq/1, Delay12/1
  V/1 -> Delay8/1, Sensitivity Calculation/8(V1)
  F/1 -> Delay10/1, Sensitivity Calculation/10(F1)
  fc/1 -> Sensitivity Calculation/1(fc)
  fc1/1 -> Average Voltage Sensitivity/1(fc)
  fc2/1 -> Average Frequency Sensitivity/1(fc)

== system STmodel_gui/PWM outputs/voltage control/Subsystem1/Triggered Subsystem ==
  In1 : Inport
  Trigger : TriggerPort  VariantControl=Variant
  Out1 : Outport
  wires:
  In1/1 -> Out1/1

== system STmodel_gui/PWM outputs/voltage control/Subsystem1/Triggered Subsystem1 ==
  In1 : Inport
  Trigger : TriggerPort  VariantControl=Variant
  Out1 : Outport
  wires:
  In1/1 -> Out1/1

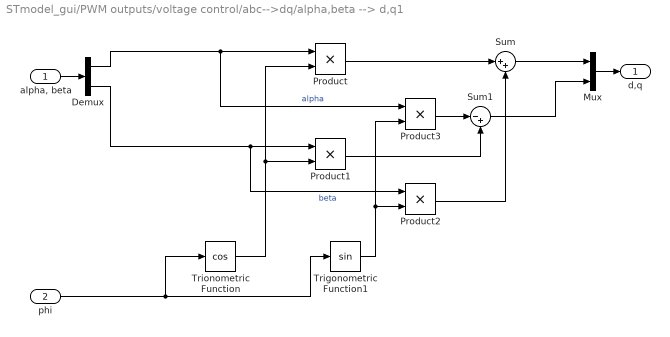
== system STmodel_gui/PWM outputs/voltage control/abc-->dq/alpha,beta --> d,q1 ==
  "alpha, beta" : Inport
  phi : Inport  Port=2
  Demux : Demux  Outputs=2
  Mux : Mux  Inputs=2
  Product{,1..3} (4 alike) : Product  RndMeth=Zero
  Sum : Sum  Inputs=|++
  Sum1 : Sum  Inputs=|-+
  Trigonometric Function1 : Trigonometry
  Trionometric Function : Trigonometry  Operator=cos
  d,q : Outport
  wires:
  "alpha, beta"/1 -> Demux/1
  Mux/1 -> d,q/1
  Demux/2 -> Product1/1, Product2/1  "beta"
  Demux/1 -> Product/1, Product3/1  "alpha"
  Trionometric Function/1 -> Product/2, Product1/2
  Trigonometric Function1/1 -> Product3/2, Product2/2
  Product/1 -> Sum/1
  Product2/1 -> Sum/2
  Sum/1 -> Mux/1
  Product3/1 -> Sum1/1
  Product1/1 -> Sum1/2
  Sum1/1 -> Mux/2
  phi/1 -> Trionometric Function/1, Trigonometric Function1/1

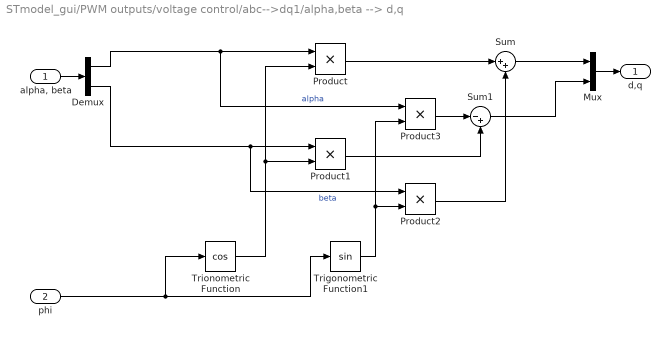
== system STmodel_gui/PWM outputs/voltage control/abc-->dq1/alpha,beta --> d,q ==
  "alpha, beta" : Inport
  phi : Inport  Port=2
  Demux : Demux  Outputs=2
  Mux : Mux  Inputs=2
  Product{,1..3} (4 alike) : Product  RndMeth=Zero
  Sum : Sum  Inputs=|++
  Sum1 : Sum  Inputs=|-+
  Trigonometric Function1 : Trigonometry
  Trionometric Function : Trigonometry  Operator=cos
  d,q : Outport
  wires:
  phi/1 -> Trigonometric Function1/1, Trionometric Function/1
  Sum1/1 -> Mux/2
  Product1/1 -> Sum1/2
  Product3/1 -> Sum1/1
  Sum/1 -> Mux/1
  Product2/1 -> Sum/2
  Product/1 -> Sum/1
  Trigonometric Function1/1 -> Product2/2, Product3/2
  Trionometric Function/1 -> Product1/2, Product/2
  Demux/1 -> Product3/1, Product/1  "alpha"
  Demux/2 -> Product2/1, Product1/1  "beta"
  Mux/1 -> d,q/1
  "alpha, beta"/1 -> Demux/1

== system STmodel_gui/PWM outputs/voltage control/abc-->dq2/alpha,beta --> d,q1 ==
  "alpha, beta" : Inport
  phi : Inport  Port=2
  Demux : Demux  Outputs=2
  Mux : Mux  Inputs=2
  Product{,1..3} (4 alike) : Product  RndMeth=Zero
  Sum : Sum  Inputs=|++
  Sum1 : Sum  Inputs=|-+
  Trigonometric Function1 : Trigonometry
  Trionometric Function : Trigonometry  Operator=cos
  d,q : Outport
  wires:
  phi/1 -> Trigonometric Function1/1, Trionometric Function/1
  Sum1/1 -> Mux/2
  Product1/1 -> Sum1/2
  Product3/1 -> Sum1/1
  Sum/1 -> Mux/1
  Product2/1 -> Sum/2
  Product/1 -> Sum/1
  Trigonometric Function1/1 -> Product2/2, Product3/2
  Trionometric Function/1 -> Product1/2, Product/2
  Demux/1 -> Product3/1, Product/1  "alpha"
  Demux/2 -> Product2/1, Product1/1  "beta"
  Mux/1 -> d,q/1
  "alpha, beta"/1 -> Demux/1

== system STmodel_gui/PWM outputs/voltage control/dq-->abc/alpha,beta --> d,q3 ==
  "d, q" : Inport
  phi : Inport  Port=2
  Demux : Demux  Outputs=2
  Mux : Mux  Inputs=2
  Product{,1..3} (4 alike) : Product  RndMeth=Zero
  Sum : Sum  Inputs=|+-
  Sum1 : Sum  Inputs=|++
  Trigonometric Function1 : Trigonometry
  Trionometric Function : Trigonometry  Operator=cos
  "alfa, beta" : Outport
  wires:
  "d, q"/1 -> Demux/1
  Mux/1 -> "alfa, beta"/1
  Demux/2 -> Product1/1, Product2/1  "q"
  Demux/1 -> Product/1, Product3/1  "d"
  Trionometric Function/1 -> Product/2, Product1/2
  Trigonometric Function1/1 -> Product3/2, Product2/2
  Product/1 -> Sum/1
  Product2/1 -> Sum/2
  Sum/1 -> Mux/1
  Product3/1 -> Sum1/1
  Product1/1 -> Sum1/2
  Sum1/1 -> Mux/2
  phi/1 -> Trionometric Function/1, Trigonometric Function1/1

== system STmodel_gui/PWM outputs/voltage control/References/Triggered Pulse Generator/singal detection ==
  note: Edge
  signal : Inport
  Delay Input1 : UnitDelay  Description=Store in Global RAM  DisableCoverage=on  SampleTime=-1  HasFrameUpgradeWarning=on
  FixPt Relational Operator : RelationalOperator  Operator=>  OutDataTypeStr=fixdt(0, 8)  ZeroCross=off  RndMeth=Nearest
  Positive : simulink/Logic and Bit Operations/Compare To Zero  relop=>  OutDataTypeStr=uint8  ZeroCross=off
  out : Outport
  wires:
  Delay Input1/1 -> FixPt Relational Operator/2  "U(k-1)"
  Positive/1 -> Delay Input1/1, FixPt Relational Operator/1  "U(k)"
  FixPt Relational Operator/1 -> out/1
  signal/1 -> Positive/1

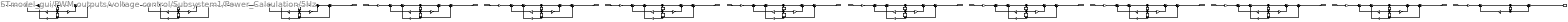
== system STmodel_gui/PWM outputs/voltage control/Subsystem1/Power_Calculation/5Hz ==
  Input : Inport
  Delay{11..19,21..29,110..113,210..212} (25 alike) : Delay  DelayLength=1  InitialCondition=0
  SumA{21..29,31..39,210..213,310..312} (25 alike) : Sum  Inputs=|+-  RndMeth=Nearest  SaturateOnIntegerOverflow=on  OutDataTypeStr=Inherit: Same as first input
  SumB{21..29,31..39,210..213,310..312} (25 alike) : Sum  Inputs=|++  RndMeth=Nearest  SaturateOnIntegerOverflow=on  OutDataTypeStr=Inherit: Same as first input
  a(2)(1) : Gain  Gain=-1.9991390072199049  ParamDataTypeStr=double  RndMeth=Nearest  SaturateOnIntegerOverflow=on  OutDataTypeStr=Inherit: Same as input
  a(2)(10) : Gain  Gain=-1.9879059014899649  ParamDataTypeStr=double  RndMeth=Nearest  SaturateOnIntegerOverflow=on  OutDataTypeStr=Inherit: Same as input
  a(2)(11) : Gain  Gain=-1.9874060536378855  ParamDataTypeStr=double  RndMeth=Nearest  SaturateOnIntegerOverflow=on  OutDataTypeStr=Inherit: Same as input
  a(2)(12) : Gain  Gain=-1.9871030789680624  ParamDataTypeStr=double  RndMeth=Nearest  SaturateOnIntegerOverflow=on  OutDataTypeStr=Inherit: Same as input
  a(2)(13) : Gain  Gain=-0.99350078718466261  ParamDataTypeStr=double  RndMeth=Nearest  SaturateOnIntegerOverflow=on  OutDataTypeStr=Inherit: Same as input
  a(2)(2) : Gain  Gain=-1.9975169417302483  ParamDataTypeStr=double  RndMeth=Nearest  SaturateOnIntegerOverflow=on  OutDataTypeStr=Inherit: Same as input
  a(2)(3) : Gain  Gain=-1.9959358866225518  ParamDataTypeStr=double  RndMeth=Nearest  SaturateOnIntegerOverflow=on  OutDataTypeStr=Inherit: Same as input
  a(2)(4) : Gain  Gain=-1.9944205297736062  ParamDataTypeStr=double  RndMeth=Nearest  SaturateOnIntegerOverflow=on  OutDataTypeStr=Inherit: Same as input
  a(2)(5) : Gain  Gain=-1.9929944232171564  ParamDataTypeStr=double  RndMeth=Nearest  SaturateOnIntegerOverflow=on  OutDataTypeStr=Inherit: Same as input
  a(2)(6) : Gain  Gain=-1.9916796336622546  ParamDataTypeStr=double  RndMeth=Nearest  SaturateOnIntegerOverflow=on  OutDataTypeStr=Inherit: Same as input
  a(2)(7) : Gain  Gain=-1.990496421142663  ParamDataTypeStr=double  RndMeth=Nearest  SaturateOnIntegerOverflow=on  OutDataTypeStr=Inherit: Same as input
  a(2)(8) : Gain  Gain=-1.9894629491880729  ParamDataTypeStr=double  RndMeth=Nearest  SaturateOnIntegerOverflow=on  OutDataTypeStr=Inherit: Same as input
  a(2)(9) : Gain  Gain=-1.9885950292459276  ParamDataTypeStr=double  RndMeth=Nearest  SaturateOnIntegerOverflow=on  OutDataTypeStr=Inherit: Same as input
  a(3)(1) : Gain  Gain=0.99918150500520764  ParamDataTypeStr=double  RndMeth=Nearest  SaturateOnIntegerOverflow=on  OutDataTypeStr=Inherit: Same as input
  a(3)(10) : Gain  Gain=0.98794816048140999  ParamDataTypeStr=double  RndMeth=Nearest  SaturateOnIntegerOverflow=on  OutDataTypeStr=Inherit: Same as input
  a(3)(11) : Gain  Gain=0.98744830200354272  ParamDataTypeStr=double  RndMeth=Nearest  SaturateOnIntegerOverflow=on  OutDataTypeStr=Inherit: Same as input
  a(3)(12) : Gain  Gain=0.98714532089307083  ParamDataTypeStr=double  RndMeth=Nearest  SaturateOnIntegerOverflow=on  OutDataTypeStr=Inherit: Same as input
  a(3)(2) : Gain  Gain=0.9975594050336114  ParamDataTypeStr=double  RndMeth=Nearest  SaturateOnIntegerOverflow=on  OutDataTypeStr=Inherit: Same as input
  a(3)(3) : Gain  Gain=0.99597831631577549  ParamDataTypeStr=double  RndMeth=Nearest  SaturateOnIntegerOverflow=on  OutDataTypeStr=Inherit: Same as input
  a(3)(4) : Gain  Gain=0.99446292725330698  ParamDataTypeStr=double  RndMeth=Nearest  SaturateOnIntegerOverflow=on  OutDataTypeStr=Inherit: Same as input
  a(3)(5) : Gain  Gain=0.99303679038062087  ParamDataTypeStr=double  RndMeth=Nearest  SaturateOnIntegerOverflow=on  OutDataTypeStr=Inherit: Same as input
  a(3)(6) : Gain  Gain=0.99172197287586472  ParamDataTypeStr=double  RndMeth=Nearest  SaturateOnIntegerOverflow=on  OutDataTypeStr=Inherit: Same as input
  a(3)(7) : Gain  Gain=0.99053873520348923  ParamDataTypeStr=double  RndMeth=Nearest  SaturateOnIntegerOverflow=on  OutDataTypeStr=Inherit: Same as input
  a(3)(8) : Gain  Gain=0.98950524127930672  ParamDataTypeStr=double  RndMeth=Nearest  SaturateOnIntegerOverflow=on  OutDataTypeStr=Inherit: Same as input
  a(3)(9) : Gain  Gain=0.9886373028868809  ParamDataTypeStr=double  RndMeth=Nearest  SaturateOnIntegerOverflow=on  OutDataTypeStr=Inherit: Same as input
  b(2)(1) : Gain  Gain=2  ParamDataTypeStr=double  RndMeth=Nearest  SaturateOnIntegerOverflow=on  OutDataTypeStr=Inherit: Same as input
  b(2)(10) : Gain  Gain=2  ParamDataTypeStr=double  RndMeth=Nearest  SaturateOnIntegerOverflow=on  OutDataTypeStr=Inherit: Same as input
  b(2)(11) : Gain  Gain=2  ParamDataTypeStr=double  RndMeth=Nearest  SaturateOnIntegerOverflow=on  OutDataTypeStr=Inherit: Same as input
  b(2)(12) : Gain  Gain=2  ParamDataTypeStr=double  RndMeth=Nearest  SaturateOnIntegerOverflow=on  OutDataTypeStr=Inherit: Same as input
  b(2)(2) : Gain  Gain=2  ParamDataTypeStr=double  RndMeth=Nearest  SaturateOnIntegerOverflow=on  OutDataTypeStr=Inherit: Same as input
  b(2)(3) : Gain  Gain=2  ParamDataTypeStr=double  RndMeth=Nearest  SaturateOnIntegerOverflow=on  OutDataTypeStr=Inherit: Same as input
  b(2)(4) : Gain  Gain=2  ParamDataTypeStr=double  RndMeth=Nearest  SaturateOnIntegerOverflow=on  OutDataTypeStr=Inherit: Same as input
  b(2)(5) : Gain  Gain=2  ParamDataTypeStr=double  RndMeth=Nearest  SaturateOnIntegerOverflow=on  OutDataTypeStr=Inherit: Same as input
  b(2)(6) : Gain  Gain=2  ParamDataTypeStr=double  RndMeth=Nearest  SaturateOnIntegerOverflow=on  OutDataTypeStr=Inherit: Same as input
  b(2)(7) : Gain  Gain=2  ParamDataTypeStr=double  RndMeth=Nearest  SaturateOnIntegerOverflow=on  OutDataTypeStr=Inherit: Same as input
  b(2)(8) : Gain  Gain=2  ParamDataTypeStr=double  RndMeth=Nearest  SaturateOnIntegerOverflow=on  OutDataTypeStr=Inherit: Same as input
  b(2)(9) : Gain  Gain=2  ParamDataTypeStr=double  RndMeth=Nearest  SaturateOnIntegerOverflow=on  OutDataTypeStr=Inherit: Same as input
  s(1) : Gain  Gain=1.0624446325651038e-05  ParamDataTypeStr=double  RndMeth=Nearest  SaturateOnIntegerOverflow=on  OutDataTypeStr=Inherit: Same as input
  s(10) : Gain  Gain=1.0564747861228558e-05  ParamDataTypeStr=double  RndMeth=Nearest  SaturateOnIntegerOverflow=on  OutDataTypeStr=Inherit: Same as input
  s(11) : Gain  Gain=1.0562091414300039e-05  ParamDataTypeStr=double  RndMeth=Nearest  SaturateOnIntegerOverflow=on  OutDataTypeStr=Inherit: Same as input
  s(12) : Gain  Gain=1.0560481252072229e-05  ParamDataTypeStr=double  RndMeth=Nearest  SaturateOnIntegerOverflow=on  OutDataTypeStr=Inherit: Same as input
  s(13) : Gain  Gain=0.0032496064076687138  ParamDataTypeStr=double  RndMeth=Nearest  SaturateOnIntegerOverflow=on  OutDataTypeStr=Inherit: Same as input
  s(2) : Gain  Gain=1.0615825840697611e-05  ParamDataTypeStr=double  RndMeth=Nearest  SaturateOnIntegerOverflow=on  OutDataTypeStr=Inherit: Same as input
  s(3) : Gain  Gain=1.0607423305871894e-05  ParamDataTypeStr=double  RndMeth=Nearest  SaturateOnIntegerOverflow=on  OutDataTypeStr=Inherit: Same as input
  s(4) : Gain  Gain=1.0599369925167656e-05  ParamDataTypeStr=double  RndMeth=Nearest  SaturateOnIntegerOverflow=on  OutDataTypeStr=Inherit: Same as input
  s(5) : Gain  Gain=1.059179086612827e-05  ParamDataTypeStr=double  RndMeth=Nearest  SaturateOnIntegerOverflow=on  OutDataTypeStr=Inherit: Same as input
  s(6) : Gain  Gain=1.0584803402522622e-05  ParamDataTypeStr=double  RndMeth=Nearest  SaturateOnIntegerOverflow=on  OutDataTypeStr=Inherit: Same as input
  s(7) : Gain  Gain=1.0578515206523825e-05  ParamDataTypeStr=double  RndMeth=Nearest  SaturateOnIntegerOverflow=on  OutDataTypeStr=Inherit: Same as input
  s(8) : Gain  Gain=1.0573022808410961e-05  ParamDataTypeStr=double  RndMeth=Nearest  SaturateOnIntegerOverflow=on  OutDataTypeStr=Inherit: Same as input
  s(9) : Gain  Gain=1.0568410238296036e-05  ParamDataTypeStr=double  RndMeth=Nearest  SaturateOnIntegerOverflow=on  OutDataTypeStr=Inherit: Same as input
  Output : Outport
  wires:
  Input/1 -> s(1)/1
  s(1)/1 -> SumA21/1
  SumA21/1 -> SumA31/1
  SumA31/1 -> SumB21/1, Delay11/1
  SumB21/1 -> SumB31/1
  SumB31/1 -> [Sect1]
  a(2)(1)/1 -> SumA21/2
  Delay11/1 -> a(2)(1)/1, b(2)(1)/1, Delay21/1
  b(2)(1)/1 -> SumB21/2
  a(3)(1)/1 -> SumA31/2
  Delay21/1 -> a(3)(1)/1, SumB31/2
  [Sect1] -> s(2)/1
  s(2)/1 -> SumA22/1
  SumA22/1 -> SumA32/1
  SumA32/1 -> SumB22/1, Delay12/1
  SumB22/1 -> SumB32/1
  SumB32/1 -> [Sect2]
  a(2)(2)/1 -> SumA22/2
  Delay12/1 -> a(2)(2)/1, b(2)(2)/1, Delay22/1
  b(2)(2)/1 -> SumB22/2
  a(3)(2)/1 -> SumA32/2
  Delay22/1 -> a(3)(2)/1, SumB32/2
  [Sect2] -> s(3)/1
  s(3)/1 -> SumA23/1
  SumA23/1 -> SumA33/1
  SumA33/1 -> SumB23/1, Delay13/1
  SumB23/1 -> SumB33/1
  SumB33/1 -> [Sect3]
  a(2)(3)/1 -> SumA23/2
  Delay13/1 -> a(2)(3)/1, b(2)(3)/1, Delay23/1
  b(2)(3)/1 -> SumB23/2
  a(3)(3)/1 -> SumA33/2
  Delay23/1 -> a(3)(3)/1, SumB33/2
  [Sect3] -> s(4)/1
  s(4)/1 -> SumA24/1
  SumA24/1 -> SumA34/1
  SumA34/1 -> SumB24/1, Delay14/1
  SumB24/1 -> SumB34/1
  SumB34/1 -> [Sect4]
  a(2)(4)/1 -> SumA24/2
  Delay14/1 -> a(2)(4)/1, b(2)(4)/1, Delay24/1
  b(2)(4)/1 -> SumB24/2
  a(3)(4)/1 -> SumA34/2
  Delay24/1 -> a(3)(4)/1, SumB34/2
  [Sect4] -> s(5)/1
  s(5)/1 -> SumA25/1
  SumA25/1 -> SumA35/1
  SumA35/1 -> SumB25/1, Delay15/1
  SumB25/1 -> SumB35/1
  SumB35/1 -> [Sect5]
  a(2)(5)/1 -> SumA25/2
  Delay15/1 -> a(2)(5)/1, b(2)(5)/1, Delay25/1
  b(2)(5)/1 -> SumB25/2
  a(3)(5)/1 -> SumA35/2
  Delay25/1 -> a(3)(5)/1, SumB35/2
  [Sect5] -> s(6)/1
  s(6)/1 -> SumA26/1
  SumA26/1 -> SumA36/1
  SumA36/1 -> SumB26/1, Delay16/1
  SumB26/1 -> SumB36/1
  SumB36/1 -> [Sect6]
  a(2)(6)/1 -> SumA26/2
  Delay16/1 -> a(2)(6)/1, b(2)(6)/1, Delay26/1
  b(2)(6)/1 -> SumB26/2
  a(3)(6)/1 -> SumA36/2
  Delay26/1 -> a(3)(6)/1, SumB36/2
  [Sect6] -> s(7)/1
  s(7)/1 -> SumA27/1
  SumA27/1 -> SumA37/1
  SumA37/1 -> SumB27/1, Delay17/1
  SumB27/1 -> SumB37/1
  SumB37/1 -> [Sect7]
  a(2)(7)/1 -> SumA27/2
  Delay17/1 -> a(2)(7)/1, b(2)(7)/1, Delay27/1
  b(2)(7)/1 -> SumB27/2
  a(3)(7)/1 -> SumA37/2
  Delay27/1 -> a(3)(7)/1, SumB37/2
  [Sect7] -> s(8)/1
  s(8)/1 -> SumA28/1
  SumA28/1 -> SumA38/1
  SumA38/1 -> SumB28/1, Delay18/1
  SumB28/1 -> SumB38/1
  SumB38/1 -> [Sect8]
  a(2)(8)/1 -> SumA28/2
  Delay18/1 -> a(2)(8)/1, b(2)(8)/1, Delay28/1
  b(2)(8)/1 -> SumB28/2
  a(3)(8)/1 -> SumA38/2
  Delay28/1 -> a(3)(8)/1, SumB38/2
  [Sect8] -> s(9)/1
  s(9)/1 -> SumA29/1
  SumA29/1 -> SumA39/1
  SumA39/1 -> SumB29/1, Delay19/1
  SumB29/1 -> SumB39/1
  SumB39/1 -> [Sect9]
  a(2)(9)/1 -> SumA29/2
  Delay19/1 -> a(2)(9)/1, b(2)(9)/1, Delay29/1
  b(2)(9)/1 -> SumB29/2
  a(3)(9)/1 -> SumA39/2
  Delay29/1 -> a(3)(9)/1, SumB39/2
  [Sect9] -> s(10)/1
  s(10)/1 -> SumA210/1
  SumA210/1 -> SumA310/1
  SumA310/1 -> SumB210/1, Delay110/1
  SumB210/1 -> SumB310/1
  SumB310/1 -> [Sect10]
  a(2)(10)/1 -> SumA210/2
  Delay110/1 -> a(2)(10)/1, b(2)(10)/1, Delay210/1
  b(2)(10)/1 -> SumB210/2
  a(3)(10)/1 -> SumA310/2
  Delay210/1 -> a(3)(10)/1, SumB310/2
  [Sect10] -> s(11)/1
  s(11)/1 -> SumA211/1
  SumA211/1 -> SumA311/1
  SumA311/1 -> SumB211/1, Delay111/1
  SumB211/1 -> SumB311/1
  SumB311/1 -> [Sect11]
  a(2)(11)/1 -> SumA211/2
  Delay111/1 -> a(2)(11)/1, b(2)(11)/1, Delay211/1
  b(2)(11)/1 -> SumB211/2
  a(3)(11)/1 -> SumA311/2
  Delay211/1 -> a(3)(11)/1, SumB311/2
  [Sect11] -> s(12)/1
  s(12)/1 -> SumA212/1
  SumA212/1 -> SumA312/1
  SumA312/1 -> SumB212/1, Delay112/1
  SumB212/1 -> SumB312/1
  SumB312/1 -> [Sect12]
  a(2)(12)/1 -> SumA212/2
  Delay112/1 -> a(2)(12)/1, b(2)(12)/1, Delay212/1
  b(2)(12)/1 -> SumB212/2
  a(3)(12)/1 -> SumA312/2
  Delay212/1 -> a(3)(12)/1, SumB312/2
  [Sect12] -> s(13)/1
  s(13)/1 -> SumA213/1
  SumA213/1 -> SumB213/1, Delay113/1
  SumB213/1 -> Output/1
  a(2)(13)/1 -> SumA213/2
  Delay113/1 -> a(2)(13)/1, SumB213/2

== matlab function STmodel_gui/PWM outputs/voltage control/References/MATLAB Function2 ==
  data: freq input; Ts input; theta output; s input
function theta = fcn(freq, Ts, s)
%#codegen
theta=s+freq*2*pi*Ts;
if (theta>2*pi)
    theta=theta-2*pi;
end

== matlab function STmodel_gui/PWM outputs/voltage control/References/MATLAB Function3 ==
  data: fc input; V output; s input; knew input
function V  = fcn(fc, s, knew)
%#codegen
    vartheta=2*0.02;
%     fc=5e3;
    
    if(knew>0)
        
    V=s-vartheta/fc;

        
    if (knew>fc/2)
        V=1-vartheta/2;
    end
    if (knew>fc*1.5)
        V=s+vartheta/fc;
    end
    if (knew>fc*2)
        V=1;
    end
%     
%     if (theta<(1-vartheta))
%         theta=theta+vartheta;
%     end
%     if (theta<=vartheta)
%     theta=1;
%     end
    else
        V=1;
    end

end

== matlab function STmodel_gui/PWM outputs/voltage control/References/MATLAB Function4 ==
  data: fc input; sign input; kold input; knewV output; flagOLD input; flagNEW output
function [knewV,flagNEW]  = fcn(fc,sign,kold,flagOLD)
%#codegen
TW=2;
% fc=5e3;


        if(sign < 0.5)
            
            knewV=0;
            flagNEW=0;

        else
           
            if(flagOLD==0)
             knewV=kold+1;
                flagNEW=0;
                if (knewV>TW*fc)
                    knewV=0;
                    flagNEW=1;
                end
            else
                knewV=0;
                flagNEW=1;
            end
        end

end

== matlab function STmodel_gui/PWM outputs/voltage control/Subsystem1/Sensitivity Calculation/Sensitivity Calculation ==
  data: fc input; knewV input; knewF input; P1 input; Kpnew output; P2 input; Q1 input; Q2 input; V1 input; V2 input; Kqnew output; F1 input; F2 input; Kfpnew output; Kfqnew output
function [Kpnew,Kqnew,Kfpnew,Kfqnew]  = fcn(fc,knewV,knewF,P1, P2, Q1, Q2, V1, V2, F1, F2)
%#codegen

%%%Time Window
TW=2;
%%%Initialization
    Kpnew = 0;
    Kqnew = 0;
    Kfpnew = 0;
    Kfqnew = 0;
    DV=0;
    DP=0;

%%% Voltage Sensitivity
DP=(P1-P2)/P2; %%% Calculation of Delta P
DQ=(Q1-Q2)/Q2;

% Calculation of single time-step of Kp and Kq
if (knewV<=0)
    Kpnew = 0;
    Kqnew = 0;

elseif(knewV>0 && knewV<fc*TW/4 || knewV>fc*TW*3/4 && knewV<fc*TW) %%% It calculates just during the voltage variation
    DV=(V1-V2)/V2;
    Kpnew = DP/DV;
    Kqnew = DQ/DV;
end

%%% Current sensitivity
if (knewF==0)
    Kfpnew = 0;
    Kfqnew = 0;
elseif(knewF>0 && knewF<fc*TW/4 || knewF>fc*TW*3/4 && knewF<fc*TW)
    DF=(F1-F2);
    Kfpnew = DP/DF;
    Kfqnew = DQ/DF;
end


end
